simulink model "MDP"  (R2017b)
settings: Solver=FixedStepDiscrete  StartTime=0.0  StopTime=Tmax  FixedStep=Ts  RelTol=1e-3
PreLoadFcn:
  | ROSconfig
  | wptsSignalSetup
PostLoadFcn:
  | config_parameters
InitFcn:
  | config_parameters
StartFcn:
  | gazeboSetup
StopFcn:
  | gazeboReset
  | goalreset
  | loadResults
model workspace (MAT data in the model file):
  MCOS : class17 (value not decoded)
  MCOS : class17 (value not decoded)
  idx = 1
  MCOS : class17 (value not decoded)
undefined symbols (not defined in the file): angmax, Angular, concDetectionAccuracy, Cthresh, DiscIntNeverNeededParam, distError, distThresh, dynamicPlume, hot, inc, init, initX, initY, Kd, Ki, Kp, Linear, mag, N, Offset, OffsetX, OffsetY, PlumeD, PlumeUpdateRate, Res, ResX, ResY, sensorDist, sourceAccuracy, T, Ts, vmax, wgain, WindX, WindY, x_g, y_g
libraries: simulink x21, dspindex x18, dspswit3 x4, robotlib x3, sm_lib x2, mobileRoboticsLib x2, nesl_utility x1, dspsnks4 x1
(part 2 of 2)

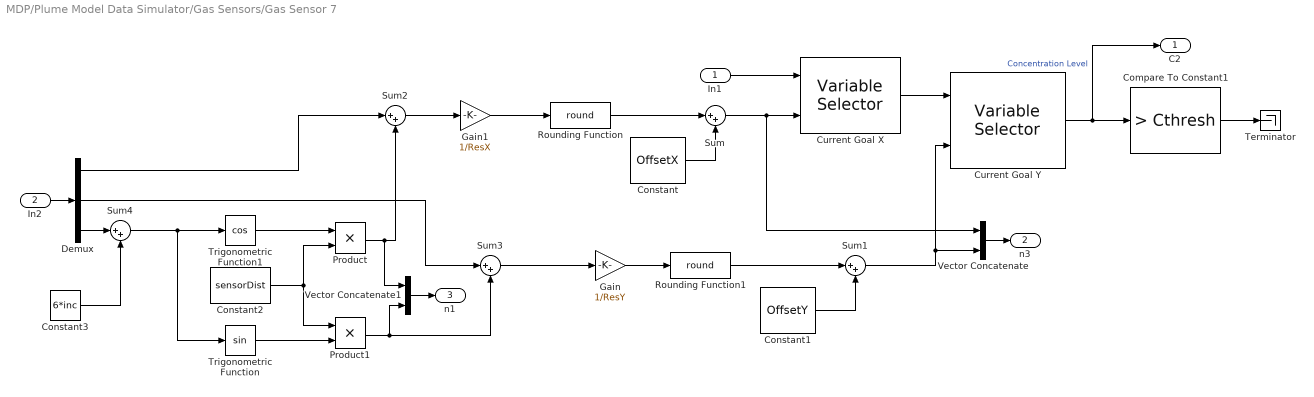
== system MDP/Plume Model Data Simulator/Gas Sensors/Gas Sensor 7 ==
  In1 : Inport
  In2 : Inport  Port=2
  Compare To Constant1 : simulink/Logic and Bit Operations/Compare To Constant  relop=>  const=Cthresh  OutDataTypeStr=boolean
  Constant : Constant  Value=OffsetX
  Constant1 : Constant  Value=OffsetY
  Constant2 : Constant  Value=sensorDist
  Constant3 : Constant  Value=6*inc
  Current Goal X : dspindex/Variable Selector  NumInputs=1  rowsOrCols=Rows  IdxMode=Variable  Elements=[1 3]  ZerOneIdxMode=One-based  errmode=Clip Index  FillMode=off  FillValues=0
  Current Goal Y : dspindex/Variable Selector  NumInputs=1  rowsOrCols=Columns  IdxMode=Variable  Elements=[1 3]  ZerOneIdxMode=One-based  errmode=Clip Index  FillMode=off  FillValues=0
  Demux : Demux  Outputs=3
  Gain : Gain  Gain=1/ResY
  Gain1 : Gain  Gain=1/ResX
  Product : Product
  Product1 : Product
  Rounding Function : Rounding  Operator=round
  Rounding Function1 : Rounding  Operator=round
  Sum{,1..4} (5 alike) : Sum  Inputs=|++
  Terminator : Terminator
  Trigonometric Function : Trigonometry
  Trigonometric Function1 : Trigonometry  Operator=cos
  Vector Concatenate : Concatenate
  Vector Concatenate1 : Concatenate
  C2 : Outport
  n3 : Outport  Port=2
  n1 : Outport  Port=3
  wires:
  In1/1 -> Current Goal X/1
  Rounding Function/1 -> Sum/1
  Current Goal Y/1 -> C2/1, Compare To Constant1/1  "Concentration Level"
  Rounding Function1/1 -> Sum1/1
  Current Goal X/1 -> Current Goal Y/1
  Constant/1 -> Sum/2
  Compare To Constant1/1 -> Terminator/1
  Constant1/1 -> Sum1/2
  Sum/1 -> Vector Concatenate/1, Current Goal X/2
  Sum1/1 -> Vector Concatenate/2, Current Goal Y/2
  Gain1/1 -> Rounding Function/1
  Gain/1 -> Rounding Function1/1
  Sum2/1 -> Gain1/1
  Sum3/1 -> Gain/1
  In2/1 -> Demux/1
  Demux/1 -> Sum2/1
  Demux/2 -> Sum3/1
  Trigonometric Function1/1 -> Product/1
  Constant2/1 -> Product1/1, Product/2
  Trigonometric Function/1 -> Product1/2
  Product/1 -> Vector Concatenate1/1, Sum2/2
  Product1/1 -> Vector Concatenate1/2, Sum3/2
  Demux/3 -> Sum4/1
  Sum4/1 -> Trigonometric Function/1, Trigonometric Function1/1
  Constant3/1 -> Sum4/2
  Vector Concatenate/1 -> n3/1
  Vector Concatenate1/1 -> n1/1

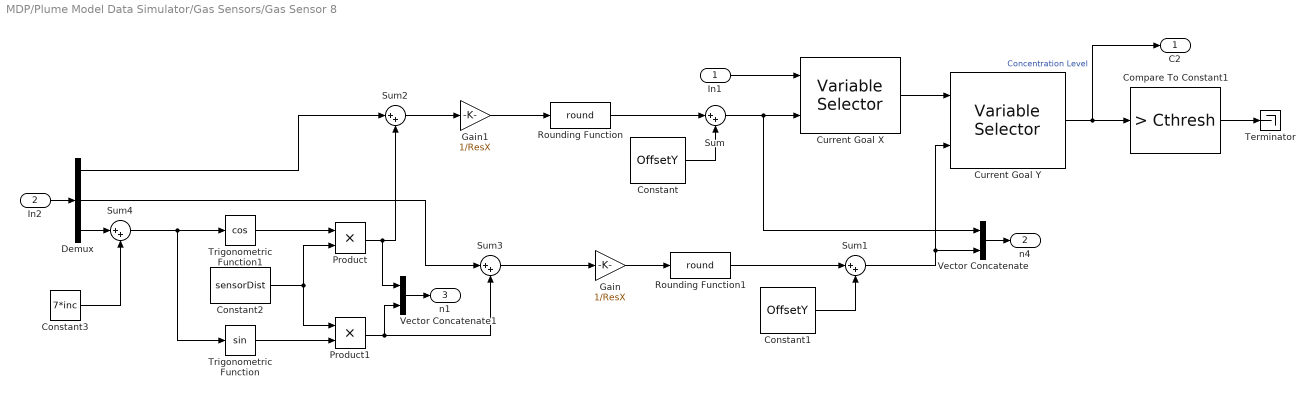
== system MDP/Plume Model Data Simulator/Gas Sensors/Gas Sensor 8 ==
  In1 : Inport
  In2 : Inport  Port=2
  Compare To Constant1 : simulink/Logic and Bit Operations/Compare To Constant  relop=>  const=Cthresh  OutDataTypeStr=boolean
  Constant : Constant  Value=OffsetY
  Constant1 : Constant  Value=OffsetY
  Constant2 : Constant  Value=sensorDist
  Constant3 : Constant  Value=7*inc
  Current Goal X : dspindex/Variable Selector  NumInputs=1  rowsOrCols=Rows  IdxMode=Variable  Elements=[1 3]  ZerOneIdxMode=One-based  errmode=Clip Index  FillMode=off  FillValues=0
  Current Goal Y : dspindex/Variable Selector  NumInputs=1  rowsOrCols=Columns  IdxMode=Variable  Elements=[1 3]  ZerOneIdxMode=One-based  errmode=Clip Index  FillMode=off  FillValues=0
  Demux : Demux  Outputs=3
  Gain : Gain  Gain=1/ResX
  Gain1 : Gain  Gain=1/ResX
  Product : Product
  Product1 : Product
  Rounding Function : Rounding  Operator=round
  Rounding Function1 : Rounding  Operator=round
  Sum{,1..4} (5 alike) : Sum  Inputs=|++
  Terminator : Terminator
  Trigonometric Function : Trigonometry
  Trigonometric Function1 : Trigonometry  Operator=cos
  Vector Concatenate : Concatenate
  Vector Concatenate1 : Concatenate
  C2 : Outport
  n4 : Outport  Port=2
  n1 : Outport  Port=3
  wires:
  In1/1 -> Current Goal X/1
  Rounding Function/1 -> Sum/1
  Current Goal Y/1 -> C2/1, Compare To Constant1/1  "Concentration Level"
  Rounding Function1/1 -> Sum1/1
  Current Goal X/1 -> Current Goal Y/1
  Constant/1 -> Sum/2
  Compare To Constant1/1 -> Terminator/1
  Constant1/1 -> Sum1/2
  Sum/1 -> Vector Concatenate/1, Current Goal X/2
  Sum1/1 -> Vector Concatenate/2, Current Goal Y/2
  Gain1/1 -> Rounding Function/1
  Gain/1 -> Rounding Function1/1
  Sum2/1 -> Gain1/1
  Sum3/1 -> Gain/1
  In2/1 -> Demux/1
  Demux/1 -> Sum2/1
  Demux/2 -> Sum3/1
  Trigonometric Function1/1 -> Product/1
  Constant2/1 -> Product1/1, Product/2
  Trigonometric Function/1 -> Product1/2
  Product/1 -> Vector Concatenate1/1, Sum2/2
  Product1/1 -> Vector Concatenate1/2, Sum3/2
  Demux/3 -> Sum4/1
  Sum4/1 -> Trigonometric Function/1, Trigonometric Function1/1
  Constant3/1 -> Sum4/2
  Vector Concatenate/1 -> n4/1
  Vector Concatenate1/1 -> n1/1

== system MDP/Plume Model Data Simulator/Gas Sensors/Gas Sensor Center ==
  In1 : Inport
  In2 : Inport  Port=2
  Compare To Constant1 : simulink/Logic and Bit Operations/Compare To Constant  relop=>  const=Cthresh  OutDataTypeStr=boolean
  Constant : Constant  Value=OffsetX
  Constant1 : Constant  Value=OffsetY
  Constant2 : Constant  Value=0
  Current Goal X : dspindex/Variable Selector  NumInputs=1  rowsOrCols=Rows  IdxMode=Variable  Elements=[1 3]  ZerOneIdxMode=One-based  errmode=Clip Index  FillMode=off  FillValues=0
  Current Goal Y : dspindex/Variable Selector  NumInputs=1  rowsOrCols=Columns  IdxMode=Variable  Elements=[1 3]  ZerOneIdxMode=One-based  errmode=Clip Index  FillMode=off  FillValues=0
  Demux : Demux  Outputs=3
  Gain : Gain  Gain=1/ResY
  Gain1 : Gain  Gain=1/ResX
  Product : Product
  Product1 : Product
  Rounding Function : Rounding  Operator=round
  Rounding Function1 : Rounding  Operator=round
  Sum{,1..3} (4 alike) : Sum  Inputs=|++
  Terminator : Terminator
  Trigonometric Function : Trigonometry
  Trigonometric Function1 : Trigonometry  Operator=cos
  Vector Concatenate : Concatenate
  C1 : Outport
  n : Outport  Port=2
  wires:
  In1/1 -> Current Goal X/1
  Rounding Function/1 -> Sum/1
  Current Goal Y/1 -> C1/1, Compare To Constant1/1  "Concentration Level"
  Rounding Function1/1 -> Sum1/1
  Current Goal X/1 -> Current Goal Y/1
  Constant/1 -> Sum/2
  Compare To Constant1/1 -> Terminator/1
  Constant1/1 -> Sum1/2
  Sum/1 -> Vector Concatenate/1, Current Goal X/2
  Sum1/1 -> Vector Concatenate/2, Current Goal Y/2
  Gain1/1 -> Rounding Function/1
  Gain/1 -> Rounding Function1/1
  Sum2/1 -> Gain1/1
  Sum3/1 -> Gain/1
  In2/1 -> Demux/1
  Demux/1 -> Sum2/1
  Demux/2 -> Sum3/1
  Demux/3 -> Trigonometric Function/1, Trigonometric Function1/1
  Constant2/1 -> Product1/1, Product/2
  Product/1 -> Sum2/2
  Product1/1 -> Sum3/2
  Vector Concatenate/1 -> n/1
  Trigonometric Function1/1 -> Product/1
  Trigonometric Function/1 -> Product1/2

== system MDP/Skill Scores/Source Estimate (SQ)/Q estimate ==
  Data Store Read : DataStoreRead  DataStoreName=Cdet
  Data Store Read1 : DataStoreRead  DataStoreName=Qest
  Data Store Read3 : DataStoreRead  DataStoreName=Qest
  Data Store Write2 : DataStoreWrite  DataStoreName=Qest
  Detect Increase : simulink/Logic and Bit Operations/Detect Increase  vinit=0.0  OutDataTypeStr=boolean
  Ground : Ground
  Relational Operator : RelationalOperator  OutDataTypeStr=boolean  RndMeth=Simplest
  Switch2 : Switch  Criteria=u2 > Threshold
  Switch3 : Switch  Criteria=u2 > Threshold
  To Workspace2 : ToWorkspace  VariableName=Qest  SaveFormat=Timeseries  SampleTime=-1
  wires:
  Ground/1 -> Switch2/3
  Detect Increase/1 -> Switch2/2
  Relational Operator/1 -> Switch3/2
  Switch2/1 -> Switch3/1, Relational Operator/1
  Data Store Read3/1 -> Switch3/3
  Switch3/1 -> To Workspace2/1, Data Store Write2/1  "Estimated Maximum"
  Data Store Read1/1 -> Relational Operator/2
  Data Store Read/1 -> Switch2/1, Detect Increase/1  "<Gas Sensor>"

== matlab function MDP/Mobile Robot Controller/Odometry Subscriber/Odom Conversion/Conversion ==
  data: yaw output; x input; y input; z input; w input
function yaw  = quat2eul(x,y,z,w)
%#codegen

% Convert the quaternion to a yaw angle (zyx euler angle)
eul = quat2eul([w,x,y,z]);
yaw = eul(1);

end

== matlab function MDP/Plume Model Data Simulator/Wind Velocities/MATLAB Function ==
  data: WindX input; WindY input; u input; WindSpeed output; WindDirection output
function [WindSpeed, WindDirection] = fcn(WindX,WindY,u)

Wx = WindX(25,25,u);
Wy = WindY(25,25,u);

WindSpeed = sqrt((Wx^2)+(Wy^2));
WindDirection = atan(Wy/Wx);

end

== matlab function MDP/Plume Model Data Simulator/Plume Concentrations/MATLAB Function ==
  data: PlumeD input; u input; Plume output; Cmax output; Peak output
function [Plume, Cmax, Peak] = fcn(PlumeD,u)

%Plume = squeeze(PlumeD(:,:,u));

Plume = PlumeD(:,:,u);

Cmax = max(max(Plume(:)));

Peak = maxmat(Plume);

end

function coord = maxmat( c )
as=size(c);
total_ele=numel(c);
[~,I]=max(c(:));
r=rem(I,as(1));
a=r;
b=((I-a)/as(1))+1;
if a==0
    a=as(1);
    b=b-1;
else
    a=r;
    b=b;
end

coord = [b,a]

end

== matlab function MDP/Subsystem1/Goal Update/goalUpdate ==
  data: pose input; goal output; ang input; mag input
function goal  = fcn(pose, ang, mag)

%xgoal = pose(1) + mag*cos(ang);
xgoal = pose(1)*4 + mag*cos(ang);
ygoal = pose(2) + mag*sin(ang);

xgoal = round(xgoal);
ygoal = round(ygoal);

goal = [xgoal,ygoal];

== matlab function MDP/MDP ==
  data: Pose input; C input; n input; ang output; N input; r input
function ang  = fcn(Pose,C,n,N,r)

fx = 0;
fy = 0;
Df = [];

% calculate the gradient at vehicle center:
for i = 1:N
    fx = fx + (C(i)-C(9))*(n(1,i))/r;
    fy = fy + (C(i)-C(9))*(n(2,i))/r;
end

fx = fx/N;
fy = fy/N;
gradf = [fx,fy];
normf = norm(gradf);

% calculate directional derivative in each search direction:
for theta = 0:(2*pi/N):2*pi
    u = [cos(theta),sin(theta)];
    Du = gradf(1)*u(1) + gradf(2)*u(2);
    Df = [Df;Du];
end

% Select the largest directional derivative and compute the heading angle
% adjustment:
Df = Df/normf;
D = find(Df == max(Df(:)));
%d = max(setdiff(Df(:),max(Df(:))));

%ang = ((pi/4)*(D(1)-1));


if isempty(D)
    ang = pi;
else
    ang = ((pi/4)*(D(1)-1));
end
%}
